simulink model "hr_smc_hybrid"  (R2024b)
settings: Solver=VariableStepAuto  StartTime=0.0  StopTime=10.0  RelTol=1e-3
values from neighbouring files (symbols this model uses):
  a = 1    [bifurcation_diagram.m]    (also in equilibria.m; flow.m; flow_analysis.m; linear_analysis.m)
  A = hr_jacobian(x_eq, a, b, d, r, s)    [params.m]
  b = 3    [bifurcation_diagram.m]    (also in equilibria.m; flow.m; flow_analysis.m; linear_analysis.m = linspace(0, 10, 100))
  c = 1    [bifurcation_diagram.m]    (also in equilibria.m; flow.m; flow_analysis.m; linear_analysis.m)
  d = 5    [bifurcation_diagram.m]    (also in equilibria.m; flow.m; flow_analysis.m; linear_analysis.m)
  I = linspace(1.2, 3.5, 1000)    [bifurcation_diagram.m]    (also in equilibria.m = 1.309; flow.m = 1.3059; linear_analysis.m = 2; params.m = 1.28)
  r = 0.003    [bifurcation_diagram.m]    (also in equilibria.m; flow.m; flow_analysis.m; linear_analysis.m = 0.001)
  s = 4    [bifurcation_diagram.m]    (also in equilibria.m; flow.m; flow_analysis.m; linear_analysis.m)
  x_r = -8/5    (= -1.6)    [bifurcation_diagram.m]    (also in equilibria.m; flow.m; flow_analysis.m; linear_analysis.m)
undefined symbols (not defined in the file or in its folder): k, x0, xd
settings Model: Creator=vincip  LastModifiedBy=vincip

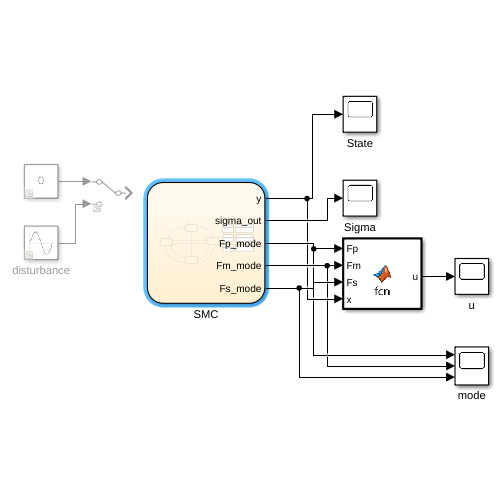
[thumbnail: Simulink's stored preview of the top-level diagram]
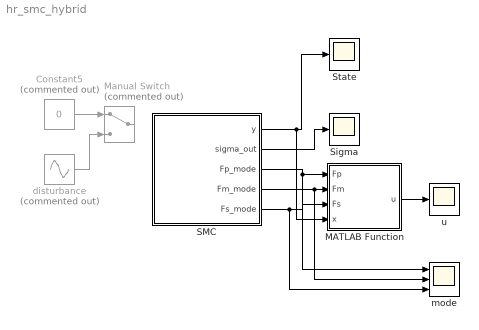
== system hr_smc_hybrid ==
  Constant5 : Constant  Commented=on  Value=0
  MATLAB Function : MATLAB Function  TreatAsAtomicUnit=on
  Manual Switch : ManualSwitch  Commented=on
  SMC : Stateflow chart  TreatAsAtomicUnit=on
  Sigma : Scope
  State : Scope
  disturbance : Sin  Commented=on  Amplitude=A  SampleTime=0
  mode : Scope  NumInputPorts=3
  u : Scope
  wires:
  SMC/1(y) -> MATLAB Function/4(x), State/1
  disturbance/1 -> Manual Switch/2
  SMC/2(sigma_out) -> Sigma/1
  Constant5/1 -> Manual Switch/1
  SMC/3(" Fp_mode") -> MATLAB Function/1(Fp), mode/1
  SMC/4(" Fm_mode") -> MATLAB Function/2(Fm), mode/2
  SMC/5(" Fs_mode") -> mode/3, MATLAB Function/3(Fs)
  MATLAB Function/1(u) -> u/1

== matlab function hr_smc_hybrid/MATLAB Function ==
  data: Fp input; u output; Fm input; Fs input; x input; a parameter; b parameter; I parameter; k parameter
function u = fcn(Fp, Fm, Fs, x, a, b, I, k)

u_eq = -x(2) + a*x(1)^3 - b*x(1)^2 + x(3) - I;

if Fp > 0
    u = u_eq - k;
elseif Fm > 0
    u = u_eq + k;
elseif Fs > 0
    u = u_eq;
else
    u = u_eq;
end

== stateflow chart hr_smc_hybrid/SMC ==
  settings: updateMethod=CONTINUOUS
  state init
    en:
    x = x_0;
    y = x;
    sigma_out = sigma;
  state Fm_mode
    during:
    x_dot = Fm;
    y = x;
    sigma_out = sigma;
  state Fp_mode
    during:
    x_dot = Fp;
    y = x;
    sigma_out = sigma;
  state Fs_mode
    during:
    x_dot = Fs;
    y = x;
    sigma_out = sigma;
  (default) -> init
  init -> Fm_mode [order 3] : [sigma < 0]
  init -> Fp_mode [order 2] : [sigma > 0]
  init -> Fs_mode [order 1] : [sigma == 0]
  Fp_mode -> Fm_mode [order 2] : [sigma <= 0 && L_sigma_Fp <= 0 && L_sigma_Fm < 0]
  Fm_mode -> Fp_mode [order 2] : [sigma >= 0 && L_sigma_Fm >= 0 && L_sigma_Fp > 0]
  Fm_mode -> Fs_mode [order 1] : [sigma >= 0 && L_sigma_Fm >= 0 && L_sigma_Fp <= 0]
  Fs_mode -> Fm_mode [order 2] : [L_sigma_Fm < 0 && L_sigma_Fp <= 0]
  Fs_mode -> Fp_mode [order 1] : [L_sigma_Fp > 0 && L_sigma_Fm >= 0]
  Fp_mode -> Fs_mode [order 1] : [sigma <= 0 && L_sigma_Fp <= 0 && L_sigma_Fm >= 0]
  data: sigma_val function_output; L_sigma_Fp_val function_output; Fp_val function_output; L_sigma_Fm_val function_output; Fm_val function_output; Fs_val function_output; x local; y output; sigma_out output; x0 parameter; xd parameter; a parameter; b parameter; c parameter; d parameter; r parameter; s parameter; x_r parameter; I parameter; k parameter; Fp_mode output boolean; Fm_mode output boolean; Fs_mode output boolean
  data x settings: updateMethod=SF_CONTINUOUS_TIME_DATA
  function sigma_val = sigma:
    | function sigma_val = sigma
    | 
    | % switching function \sigma(x) = p^T(x - xd)
    | sigma_val = (x(1) - xd);
  function L_sigma_Fp_val = L_sigma_Fp:
    | function L_sigma_Fp_val = L_sigma_Fp
    | 
    | %Lie derivative of sigma wrt Fp
    | L_sigma_Fp_val = [1 0 0] * Fp;
  function Fp_val = Fp:
    | function Fp_val = Fp
    | 
    | % equivalent control
    | u_eq = -x(2) + a*x(1)^3 - b*x(1)^2 + x(3) - I;
    | % switching control
    | u_sw = - k;
    | 
    | % cumulative control action
    | u = u_eq + u_sw;
    | 
    | % vector field Fp
    | Fp_val = [x(2) - a*x(1)^3 + b*x(1)^2 - x(3) + I + u;...
    |             c - d*x(1)^2 - x(2);...
    |             r*(s*(x(1) - x_r) - x(3));];
  function L_sigma_Fm_val = L_sigma_Fm:
    | function L_sigma_Fm_val = L_sigma_Fm
    | 
    | %Lie derivative of sigma wrt Fm
    | L_sigma_Fm_val = [1 0 0] * Fm;
  function Fm_val = Fm:
    | function Fm_val = Fm
    | 
    | % equivalent control
    | u_eq = -x(2) + a*x(1)^3 - b*x(1)^2 + x(3) - I;
    | 
    | % switching control
    | u_sw = + k;
    | 
    | % cumulative control
    | u = u_eq + u_sw;
    | 
    | % vector field Fm
    | Fm_val = [x(2) - a*x(1)^3 + b*x(1)^2 - x(3) + I + u;...
    |             c - d*x(1)^2 - x(2);...
    |             r*(s*(x(1) - x_r) - x(3));];
  function Fs_val = Fs:
    | function Fs_val = Fs
    | 
    | % derivation of the sliding vector field via convexification method
    | 
    | alpha = L_sigma_Fp / (L_sigma_Fp - L_sigma_Fm);
    | 
    | Fs_val = alpha * Fm + (1 - alpha) * Fp;
